simulink library "inSOMANET"  (R2016b)
settings: Solver=VariableStepAuto  StartTime=0.0  StopTime=10.0  RelTol=1e-3
undefined symbols (not defined in the file): jointPolarityLHFE, jointPolarityLKFE, jointPolarityRHFE, jointPolarityRKFE, resolutionJointEncoder, resolutionMotorEncoder, torquePolarityLHFE, torquePolarityLKFE, torquePolarityRHFE, torquePolarityRKFE, zeroOffsetLHFE, zeroOffsetLKFE, zeroOffsetRHFE, zeroOffsetRKFE
libraries: xpcethercatlib x70, ConversionsLibrary x64, simulink_extras x8
settings Model: Creator=Nathan  LastModifiedBy=march

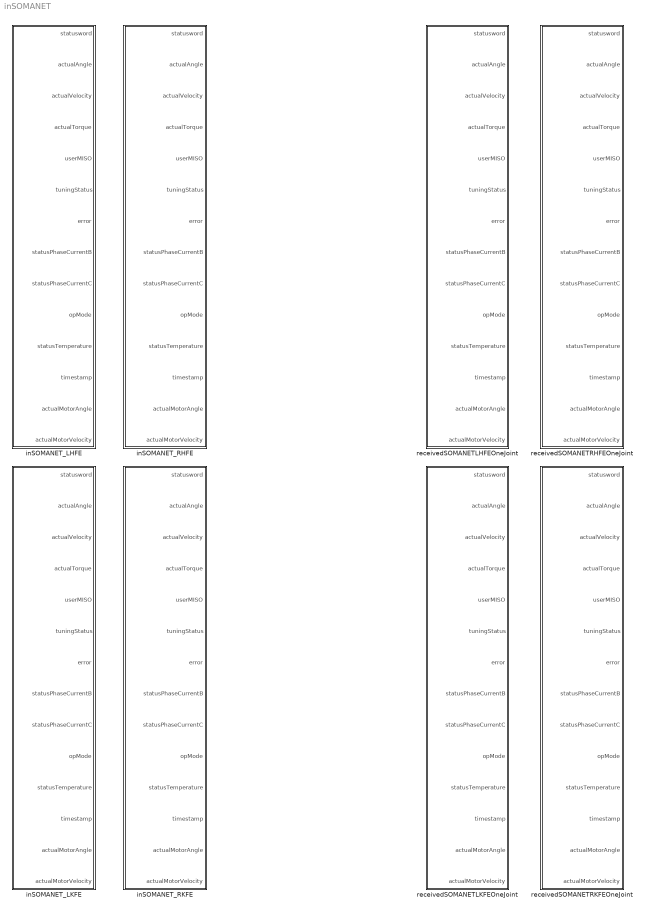
== system inSOMANET ==
  inSOMANET_LHFE : Subsystem
  inSOMANET_LKFE : Subsystem
  inSOMANET_RHFE : Subsystem
  inSOMANET_RKFE : Subsystem
  receivedSOMANETLHFEOneJoint : Subsystem
  receivedSOMANETLKFEOneJoint : Subsystem
  receivedSOMANETRHFEOneJoint : Subsystem
  receivedSOMANETRKFEOneJoint : Subsystem

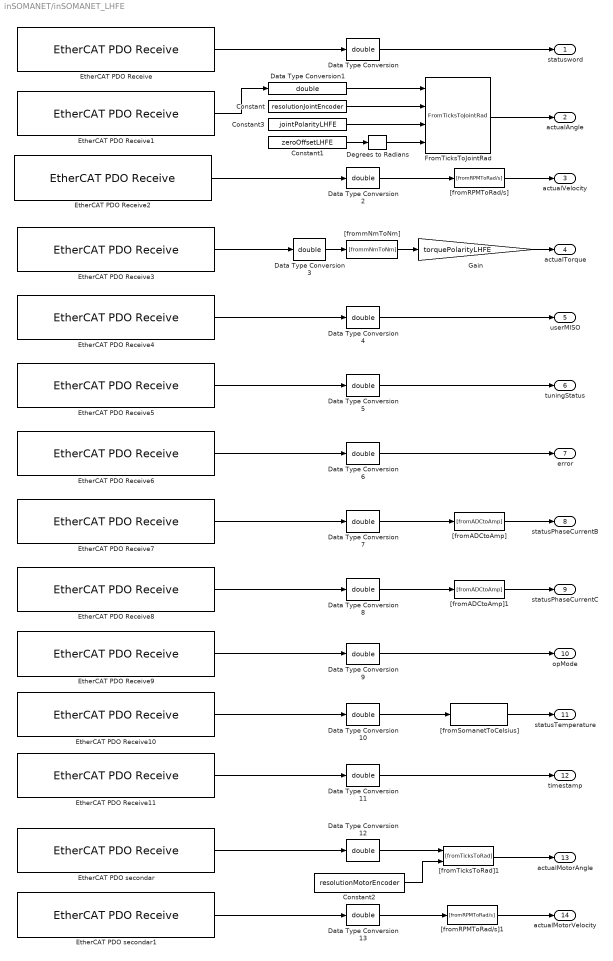
== system inSOMANET/inSOMANET_LHFE ==
  Constant : Constant  Value=resolutionJointEncoder
  Constant1 : Constant  Value=zeroOffsetLHFE  SampleTime=-1
  Constant2 : Constant  Value=resolutionMotorEncoder
  Constant3 : Constant  Value=jointPolarityLHFE
  Data Type Conversion{,1..13} (14 alike) : DataTypeConversion  OutDataTypeStr=double
  Degrees to Radians : simulink_extras/Transformations/Degrees to Radians
  EtherCAT PDO Receive : xpcethercatlib/EtherCAT PDO Receive  Priority=2  sig_name=Drive 1 LHFE.Inputs.Statusword  sig_offset=208  sig_type=uint16  type_size=16  sig_dim=1  device_id=0  sample_time=0.002000
  EtherCAT PDO Receive1 : xpcethercatlib/EtherCAT PDO Receive  Priority=2  sig_name=Drive 1 LHFE.Inputs.Position Value  sig_offset=232  sig_type=int32  type_size=32  sig_dim=1  device_id=0  sample_time=0.002000
  EtherCAT PDO Receive10 : xpcethercatlib/EtherCAT PDO Receive  Priority=2  sig_name=Drive 1 LHFE.Inputs.Core Temp  sig_offset=616  sig_type=int16  type_size=16  sig_dim=1  device_id=0  sample_time=0.002000
  EtherCAT PDO Receive11 : xpcethercatlib/EtherCAT PDO Receive  Priority=2  sig_name=Drive 1 LHFE.Inputs.timestamp  sig_offset=536  sig_type=uint32  type_size=32  sig_dim=1  device_id=0  sample_time=0.002000
  EtherCAT PDO Receive2 : xpcethercatlib/EtherCAT PDO Receive  Priority=2  sig_name=Drive 1 LHFE.Inputs.Velocity Value  sig_offset=264  sig_type=int32  type_size=32  sig_dim=1  device_id=0  sample_time=0.002000
  EtherCAT PDO Receive3 : xpcethercatlib/EtherCAT PDO Receive  Priority=2  sig_name=Drive 1 LHFE.Inputs.Torque Value  sig_offset=296  sig_type=int16  type_size=16  sig_dim=1  device_id=0  sample_time=0.002000
  EtherCAT PDO Receive4 : xpcethercatlib/EtherCAT PDO Receive  Priority=2  sig_name=Drive 1 LHFE.Inputs.User MISO  sig_offset=504  sig_type=uint32  type_size=32  sig_dim=1  device_id=0  sample_time=0.002000
  EtherCAT PDO Receive5 : xpcethercatlib/EtherCAT PDO Receive  Priority=2  sig_name=Drive 1 LHFE.Inputs.Tuning status  sig_offset=440  sig_type=uint32  type_size=32  sig_dim=1  device_id=0  sample_time=0.002000
  EtherCAT PDO Receive6 : xpcethercatlib/EtherCAT PDO Receive  Priority=2  sig_name=Drive 1 LHFE.Inputs.Error code  sig_offset=568  sig_type=uint16  type_size=16  sig_dim=1  device_id=0  sample_time=0.002000
  EtherCAT PDO Receive7 : xpcethercatlib/EtherCAT PDO Receive  Priority=2  sig_name=Drive 1 LHFE.Inputs.Phase B  sig_offset=584  sig_type=int16  type_size=16  sig_dim=1  device_id=0  sample_time=0.002000
  EtherCAT PDO Receive8 : xpcethercatlib/EtherCAT PDO Receive  Priority=2  sig_name=Drive 1 LHFE.Inputs.Phase C  sig_offset=600  sig_type=int16  type_size=16  sig_dim=1  device_id=0  sample_time=0.002000
  EtherCAT PDO Receive9 : xpcethercatlib/EtherCAT PDO Receive  Priority=2  sig_name=Drive 1 LHFE.Inputs.Op Mode Display  sig_offset=224  sig_type=int8  type_size=8  sig_dim=1  device_id=0  sample_time=0.002000
  EtherCAT PDO secondar : xpcethercatlib/EtherCAT PDO Receive  Priority=2  sig_name=Drive 1 LHFE.Inputs.Secondary position value  sig_offset=312  sig_type=int32  type_size=32  sig_dim=1  device_id=0  sample_time=0.002000
  EtherCAT PDO secondar1 : xpcethercatlib/EtherCAT PDO Receive  Priority=2  sig_name=Drive 1 LHFE.Inputs.Secondary velocity value  sig_offset=344  sig_type=int32  type_size=32  sig_dim=1  device_id=0  sample_time=0.002000
  FromTicksToJointRad : ConversionsLibrary/FromTicksToJointRad
  Gain : Gain  Gain=torquePolarityLHFE
  "[fromADCtoAmp]" : ConversionsLibrary/[fromADCtoAmp]
  "[fromADCtoAmp]1" : ConversionsLibrary/[fromADCtoAmp]
  "[fromRPMToRad/s]" : ConversionsLibrary/[fromRPMToRad//s]
  "[fromRPMToRad/s]1" : ConversionsLibrary/[fromRPMToRad//s]
  "[fromSomanetToCelsius]" : ConversionsLibrary/[fromSomanetToCelsius]
  "[fromTicksToRad]1" : ConversionsLibrary/[fromTicksToRad]
  "[frommNmToNm]" : ConversionsLibrary/[frommNmToNm]
  statusword : Outport
  actualAngle : Outport  Port=2
  actualVelocity : Outport  Port=3
  actualTorque : Outport  Port=4
  userMISO : Outport  Port=5
  tuningStatus : Outport  Port=6
  error : Outport  Port=7
  statusPhaseCurrentB : Outport  Port=8
  statusPhaseCurrentC : Outport  Port=9
  opMode : Outport  Port=10
  statusTemperature : Outport  Port=11
  timestamp : Outport  Port=12
  actualMotorAngle : Outport  Port=13
  actualMotorVelocity : Outport  Port=14
  wires:
  EtherCAT PDO secondar1/1 -> Data Type Conversion13/1
  Data Type Conversion13/1 -> "[fromRPMToRad/s]1"/1
  EtherCAT PDO secondar/1 -> Data Type Conversion12/1
  EtherCAT PDO Receive11/1 -> Data Type Conversion11/1
  EtherCAT PDO Receive10/1 -> Data Type Conversion10/1
  EtherCAT PDO Receive9/1 -> Data Type Conversion9/1
  EtherCAT PDO Receive8/1 -> Data Type Conversion8/1
  EtherCAT PDO Receive7/1 -> Data Type Conversion7/1
  EtherCAT PDO Receive6/1 -> Data Type Conversion6/1
  EtherCAT PDO Receive5/1 -> Data Type Conversion5/1
  EtherCAT PDO Receive4/1 -> Data Type Conversion4/1
  EtherCAT PDO Receive3/1 -> Data Type Conversion3/1
  EtherCAT PDO Receive2/1 -> Data Type Conversion2/1
  EtherCAT PDO Receive1/1 -> Data Type Conversion1/1
  EtherCAT PDO Receive/1 -> Data Type Conversion/1
  Data Type Conversion/1 -> statusword/1
  Data Type Conversion10/1 -> "[fromSomanetToCelsius]"/1
  Data Type Conversion9/1 -> opMode/1
  Data Type Conversion8/1 -> "[fromADCtoAmp]1"/1
  Data Type Conversion7/1 -> "[fromADCtoAmp]"/1
  Data Type Conversion6/1 -> error/1
  Data Type Conversion5/1 -> tuningStatus/1
  Data Type Conversion4/1 -> userMISO/1
  Data Type Conversion3/1 -> "[frommNmToNm]"/1
  Data Type Conversion2/1 -> "[fromRPMToRad/s]"/1
  Data Type Conversion11/1 -> timestamp/1
  "[fromSomanetToCelsius]"/1 -> statusTemperature/1
  "[fromADCtoAmp]1"/1 -> statusPhaseCurrentC/1
  "[fromADCtoAmp]"/1 -> statusPhaseCurrentB/1
  "[frommNmToNm]"/1 -> Gain/1
  "[fromRPMToRad/s]"/1 -> actualVelocity/1
  Constant1/1 -> Degrees to Radians/1
  FromTicksToJointRad/1 -> actualAngle/1
  Data Type Conversion12/1 -> "[fromTicksToRad]1"/1
  "[fromTicksToRad]1"/1 -> actualMotorAngle/1
  Constant2/1 -> "[fromTicksToRad]1"/2
  "[fromRPMToRad/s]1"/1 -> actualMotorVelocity/1
  Degrees to Radians/1 -> FromTicksToJointRad/4
  Data Type Conversion1/1 -> FromTicksToJointRad/1
  Constant/1 -> FromTicksToJointRad/2
  Constant3/1 -> FromTicksToJointRad/3
  Gain/1 -> actualTorque/1

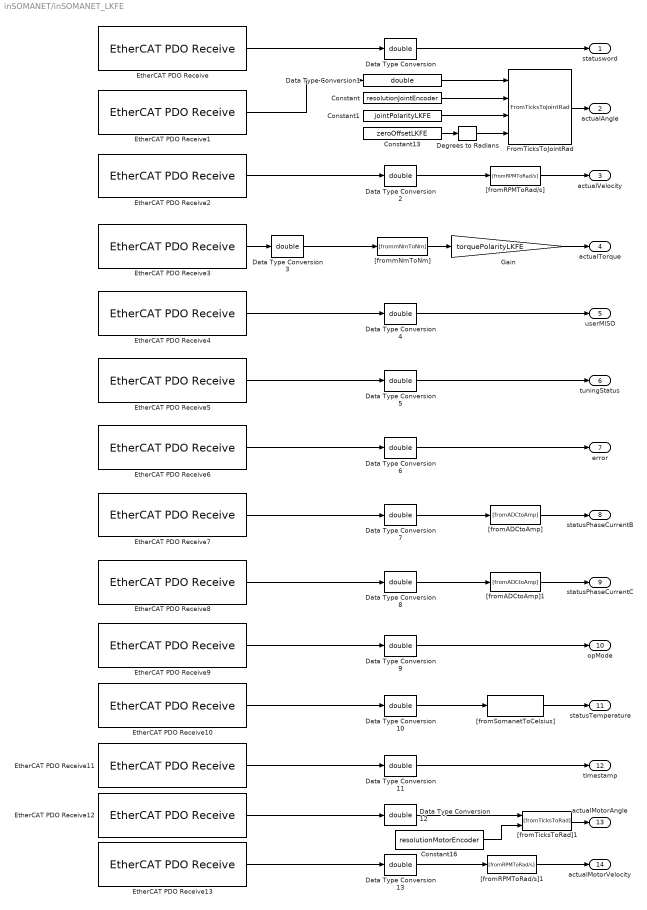
== system inSOMANET/inSOMANET_LKFE ==
  Constant : Constant  Value=resolutionJointEncoder
  Constant1 : Constant  Value=jointPolarityLKFE
  Constant13 : Constant  Value=zeroOffsetLKFE  SampleTime=-1
  Constant16 : Constant  Value=resolutionMotorEncoder
  Data Type Conversion{,1..13} (14 alike) : DataTypeConversion  OutDataTypeStr=double
  Degrees to Radians : simulink_extras/Transformations/Degrees to Radians
  EtherCAT PDO Receive : xpcethercatlib/EtherCAT PDO Receive  Priority=2  sig_name=Drive 2 LKFE.Inputs.Statusword  sig_offset=632  sig_type=uint16  type_size=16  sig_dim=1  device_id=0  sample_time=0.002000
  EtherCAT PDO Receive1 : xpcethercatlib/EtherCAT PDO Receive  Priority=2  sig_name=Drive 2 LKFE.Inputs.Position Value  sig_offset=656  sig_type=int32  type_size=32  sig_dim=1  device_id=0  sample_time=0.002000
  EtherCAT PDO Receive10 : xpcethercatlib/EtherCAT PDO Receive  Priority=2  sig_name=Drive 2 LKFE.Inputs.Core Temp  sig_offset=1040  sig_type=int16  type_size=16  sig_dim=1  device_id=0  sample_time=0.002000
  EtherCAT PDO Receive11 : xpcethercatlib/EtherCAT PDO Receive  Priority=2  sig_name=Drive 2 LKFE.Inputs.timestamp  sig_offset=960  sig_type=uint32  type_size=32  sig_dim=1  device_id=0  sample_time=0.002000
  EtherCAT PDO Receive12 : xpcethercatlib/EtherCAT PDO Receive  Priority=2  sig_name=Drive 2 LKFE.Inputs.Secondary position value  sig_offset=736  sig_type=int32  type_size=32  sig_dim=1  device_id=0  sample_time=0.002000
  EtherCAT PDO Receive13 : xpcethercatlib/EtherCAT PDO Receive  Priority=2  sig_name=Drive 2 LKFE.Inputs.Secondary velocity value  sig_offset=768  sig_type=int32  type_size=32  sig_dim=1  device_id=0  sample_time=0.002000
  EtherCAT PDO Receive2 : xpcethercatlib/EtherCAT PDO Receive  Priority=2  sig_name=Drive 2 LKFE.Inputs.Velocity Value  sig_offset=688  sig_type=int32  type_size=32  sig_dim=1  device_id=0  sample_time=0.002000
  EtherCAT PDO Receive3 : xpcethercatlib/EtherCAT PDO Receive  Priority=2  sig_name=Drive 2 LKFE.Inputs.Torque Value  sig_offset=720  sig_type=int16  type_size=16  sig_dim=1  device_id=0  sample_time=0.002000
  EtherCAT PDO Receive4 : xpcethercatlib/EtherCAT PDO Receive  Priority=2  sig_name=Drive 2 LKFE.Inputs.User MISO  sig_offset=928  sig_type=uint32  type_size=32  sig_dim=1  device_id=0  sample_time=0.002000
  EtherCAT PDO Receive5 : xpcethercatlib/EtherCAT PDO Receive  Priority=2  sig_name=Drive 2 LKFE.Inputs.Tuning status  sig_offset=864  sig_type=uint32  type_size=32  sig_dim=1  device_id=0  sample_time=0.002000
  EtherCAT PDO Receive6 : xpcethercatlib/EtherCAT PDO Receive  Priority=2  sig_name=Drive 2 LKFE.Inputs.Error code  sig_offset=992  sig_type=uint16  type_size=16  sig_dim=1  device_id=0  sample_time=0.002000
  EtherCAT PDO Receive7 : xpcethercatlib/EtherCAT PDO Receive  Priority=2  sig_name=Drive 2 LKFE.Inputs.Phase B  sig_offset=1008  sig_type=int16  type_size=16  sig_dim=1  device_id=0  sample_time=0.002000
  EtherCAT PDO Receive8 : xpcethercatlib/EtherCAT PDO Receive  Priority=2  sig_name=Drive 2 LKFE.Inputs.Phase C  sig_offset=1024  sig_type=int16  type_size=16  sig_dim=1  device_id=0  sample_time=0.002000
  EtherCAT PDO Receive9 : xpcethercatlib/EtherCAT PDO Receive  Priority=2  sig_name=Drive 2 LKFE.Inputs.Op Mode Display  sig_offset=648  sig_type=int8  type_size=8  sig_dim=1  device_id=0  sample_time=0.002000
  FromTicksToJointRad : ConversionsLibrary/FromTicksToJointRad
  Gain : Gain  Gain=torquePolarityLKFE
  "[fromADCtoAmp]" : ConversionsLibrary/[fromADCtoAmp]
  "[fromADCtoAmp]1" : ConversionsLibrary/[fromADCtoAmp]
  "[fromRPMToRad/s]" : ConversionsLibrary/[fromRPMToRad//s]
  "[fromRPMToRad/s]1" : ConversionsLibrary/[fromRPMToRad//s]
  "[fromSomanetToCelsius]" : ConversionsLibrary/[fromSomanetToCelsius]
  "[fromTicksToRad]1" : ConversionsLibrary/[fromTicksToRad]
  "[frommNmToNm]" : ConversionsLibrary/[frommNmToNm]
  statusword : Outport
  actualAngle : Outport  Port=2
  actualVelocity : Outport  Port=3
  actualTorque : Outport  Port=4
  userMISO : Outport  Port=5
  tuningStatus : Outport  Port=6
  error : Outport  Port=7
  statusPhaseCurrentB : Outport  Port=8
  statusPhaseCurrentC : Outport  Port=9
  opMode : Outport  Port=10
  statusTemperature : Outport  Port=11
  timestamp : Outport  Port=12
  actualMotorAngle : Outport  Port=13
  actualMotorVelocity : Outport  Port=14
  wires:
  EtherCAT PDO Receive13/1 -> Data Type Conversion13/1
  Data Type Conversion13/1 -> "[fromRPMToRad/s]1"/1
  EtherCAT PDO Receive12/1 -> Data Type Conversion12/1
  EtherCAT PDO Receive11/1 -> Data Type Conversion11/1
  EtherCAT PDO Receive10/1 -> Data Type Conversion10/1
  EtherCAT PDO Receive9/1 -> Data Type Conversion9/1
  EtherCAT PDO Receive8/1 -> Data Type Conversion8/1
  EtherCAT PDO Receive7/1 -> Data Type Conversion7/1
  EtherCAT PDO Receive6/1 -> Data Type Conversion6/1
  EtherCAT PDO Receive5/1 -> Data Type Conversion5/1
  EtherCAT PDO Receive4/1 -> Data Type Conversion4/1
  EtherCAT PDO Receive3/1 -> Data Type Conversion3/1
  EtherCAT PDO Receive2/1 -> Data Type Conversion2/1
  EtherCAT PDO Receive1/1 -> Data Type Conversion1/1
  EtherCAT PDO Receive/1 -> Data Type Conversion/1
  Data Type Conversion/1 -> statusword/1
  Data Type Conversion10/1 -> "[fromSomanetToCelsius]"/1
  Data Type Conversion9/1 -> opMode/1
  Data Type Conversion8/1 -> "[fromADCtoAmp]1"/1
  Data Type Conversion7/1 -> "[fromADCtoAmp]"/1
  Data Type Conversion6/1 -> error/1
  Data Type Conversion5/1 -> tuningStatus/1
  Data Type Conversion4/1 -> userMISO/1
  Data Type Conversion3/1 -> "[frommNmToNm]"/1
  Data Type Conversion2/1 -> "[fromRPMToRad/s]"/1
  Data Type Conversion11/1 -> timestamp/1
  "[fromSomanetToCelsius]"/1 -> statusTemperature/1
  "[fromADCtoAmp]1"/1 -> statusPhaseCurrentC/1
  "[fromADCtoAmp]"/1 -> statusPhaseCurrentB/1
  "[frommNmToNm]"/1 -> Gain/1
  "[fromRPMToRad/s]"/1 -> actualVelocity/1
  Constant13/1 -> Degrees to Radians/1
  Constant16/1 -> "[fromTicksToRad]1"/2
  "[fromTicksToRad]1"/1 -> actualMotorAngle/1
  Data Type Conversion12/1 -> "[fromTicksToRad]1"/1
  "[fromRPMToRad/s]1"/1 -> actualMotorVelocity/1
  Degrees to Radians/1 -> FromTicksToJointRad/4
  Constant/1 -> FromTicksToJointRad/2
  Data Type Conversion1/1 -> FromTicksToJointRad/1
  Constant1/1 -> FromTicksToJointRad/3
  FromTicksToJointRad/1 -> actualAngle/1
  Gain/1 -> actualTorque/1

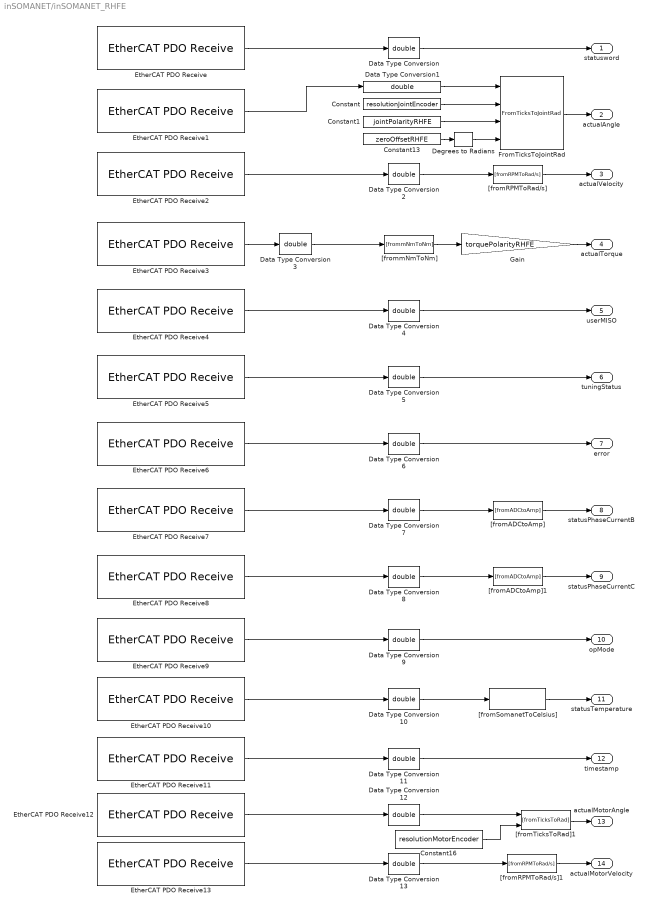
== system inSOMANET/inSOMANET_RHFE ==
  Constant : Constant  Value=resolutionJointEncoder
  Constant1 : Constant  Value=jointPolarityRHFE
  Constant13 : Constant  Value=zeroOffsetRHFE  SampleTime=-1
  Constant16 : Constant  Value=resolutionMotorEncoder
  Data Type Conversion{,1..13} (14 alike) : DataTypeConversion  OutDataTypeStr=double
  Degrees to Radians : simulink_extras/Transformations/Degrees to Radians
  EtherCAT PDO Receive : xpcethercatlib/EtherCAT PDO Receive  Priority=2  sig_name=Drive 3 RHFE.Inputs.Statusword  sig_offset=1056  sig_type=uint16  type_size=16  sig_dim=1  device_id=0  sample_time=0.002000
  EtherCAT PDO Receive1 : xpcethercatlib/EtherCAT PDO Receive  Priority=2  sig_name=Drive 3 RHFE.Inputs.Position Value  sig_offset=1080  sig_type=int32  type_size=32  sig_dim=1  device_id=0  sample_time=0.002000
  EtherCAT PDO Receive10 : xpcethercatlib/EtherCAT PDO Receive  Priority=2  sig_name=Drive 3 RHFE.Inputs.Core Temp  sig_offset=1464  sig_type=int16  type_size=16  sig_dim=1  device_id=0  sample_time=0.002000
  EtherCAT PDO Receive11 : xpcethercatlib/EtherCAT PDO Receive  Priority=2  sig_name=Drive 3 RHFE.Inputs.timestamp  sig_offset=1384  sig_type=uint32  type_size=32  sig_dim=1  device_id=0  sample_time=0.002000
  EtherCAT PDO Receive12 : xpcethercatlib/EtherCAT PDO Receive  Priority=2  sig_name=Drive 3 RHFE.Inputs.Secondary position value  sig_offset=1160  sig_type=int32  type_size=32  sig_dim=1  device_id=0  sample_time=0.002000
  EtherCAT PDO Receive13 : xpcethercatlib/EtherCAT PDO Receive  Priority=2  sig_name=Drive 3 RHFE.Inputs.Secondary velocity value  sig_offset=1192  sig_type=int32  type_size=32  sig_dim=1  device_id=0  sample_time=0.002000
  EtherCAT PDO Receive2 : xpcethercatlib/EtherCAT PDO Receive  Priority=2  sig_name=Drive 3 RHFE.Inputs.Velocity Value  sig_offset=1112  sig_type=int32  type_size=32  sig_dim=1  device_id=0  sample_time=0.002000
  EtherCAT PDO Receive3 : xpcethercatlib/EtherCAT PDO Receive  Priority=2  sig_name=Drive 3 RHFE.Inputs.Torque Value  sig_offset=1144  sig_type=int16  type_size=16  sig_dim=1  device_id=0  sample_time=0.002000
  EtherCAT PDO Receive4 : xpcethercatlib/EtherCAT PDO Receive  Priority=2  sig_name=Drive 3 RHFE.Inputs.User MISO  sig_offset=1352  sig_type=uint32  type_size=32  sig_dim=1  device_id=0  sample_time=0.002000
  EtherCAT PDO Receive5 : xpcethercatlib/EtherCAT PDO Receive  Priority=2  sig_name=Drive 3 RHFE.Inputs.Tuning status  sig_offset=1288  sig_type=uint32  type_size=32  sig_dim=1  device_id=0  sample_time=0.002000
  EtherCAT PDO Receive6 : xpcethercatlib/EtherCAT PDO Receive  Priority=2  sig_name=Drive 3 RHFE.Inputs.Error code  sig_offset=1416  sig_type=uint16  type_size=16  sig_dim=1  device_id=0  sample_time=0.002000
  EtherCAT PDO Receive7 : xpcethercatlib/EtherCAT PDO Receive  Priority=2  sig_name=Drive 3 RHFE.Inputs.Phase B  sig_offset=1432  sig_type=int16  type_size=16  sig_dim=1  device_id=0  sample_time=0.002000
  EtherCAT PDO Receive8 : xpcethercatlib/EtherCAT PDO Receive  Priority=2  sig_name=Drive 3 RHFE.Inputs.Phase C  sig_offset=1448  sig_type=int16  type_size=16  sig_dim=1  device_id=0  sample_time=0.002000
  EtherCAT PDO Receive9 : xpcethercatlib/EtherCAT PDO Receive  Priority=2  sig_name=Drive 3 RHFE.Inputs.Op Mode Display  sig_offset=1072  sig_type=int8  type_size=8  sig_dim=1  device_id=0  sample_time=0.002000
  FromTicksToJointRad : ConversionsLibrary/FromTicksToJointRad
  Gain : Gain  Gain=torquePolarityRHFE
  "[fromADCtoAmp]" : ConversionsLibrary/[fromADCtoAmp]
  "[fromADCtoAmp]1" : ConversionsLibrary/[fromADCtoAmp]
  "[fromRPMToRad/s]" : ConversionsLibrary/[fromRPMToRad//s]
  "[fromRPMToRad/s]1" : ConversionsLibrary/[fromRPMToRad//s]
  "[fromSomanetToCelsius]" : ConversionsLibrary/[fromSomanetToCelsius]
  "[fromTicksToRad]1" : ConversionsLibrary/[fromTicksToRad]
  "[frommNmToNm]" : ConversionsLibrary/[frommNmToNm]
  statusword : Outport
  actualAngle : Outport  Port=2
  actualVelocity : Outport  Port=3
  actualTorque : Outport  Port=4
  userMISO : Outport  Port=5
  tuningStatus : Outport  Port=6
  error : Outport  Port=7
  statusPhaseCurrentB : Outport  Port=8
  statusPhaseCurrentC : Outport  Port=9
  opMode : Outport  Port=10
  statusTemperature : Outport  Port=11
  timestamp : Outport  Port=12
  actualMotorAngle : Outport  Port=13
  actualMotorVelocity : Outport  Port=14
  wires:
  EtherCAT PDO Receive13/1 -> Data Type Conversion13/1
  Data Type Conversion13/1 -> "[fromRPMToRad/s]1"/1
  EtherCAT PDO Receive12/1 -> Data Type Conversion12/1
  EtherCAT PDO Receive11/1 -> Data Type Conversion11/1
  EtherCAT PDO Receive10/1 -> Data Type Conversion10/1
  EtherCAT PDO Receive9/1 -> Data Type Conversion9/1
  EtherCAT PDO Receive8/1 -> Data Type Conversion8/1
  EtherCAT PDO Receive7/1 -> Data Type Conversion7/1
  EtherCAT PDO Receive6/1 -> Data Type Conversion6/1
  EtherCAT PDO Receive5/1 -> Data Type Conversion5/1
  EtherCAT PDO Receive4/1 -> Data Type Conversion4/1
  EtherCAT PDO Receive3/1 -> Data Type Conversion3/1
  EtherCAT PDO Receive2/1 -> Data Type Conversion2/1
  EtherCAT PDO Receive1/1 -> Data Type Conversion1/1
  EtherCAT PDO Receive/1 -> Data Type Conversion/1
  Data Type Conversion/1 -> statusword/1
  Data Type Conversion10/1 -> "[fromSomanetToCelsius]"/1
  Data Type Conversion9/1 -> opMode/1
  Data Type Conversion8/1 -> "[fromADCtoAmp]1"/1
  Data Type Conversion7/1 -> "[fromADCtoAmp]"/1
  Data Type Conversion6/1 -> error/1
  Data Type Conversion5/1 -> tuningStatus/1
  Data Type Conversion4/1 -> userMISO/1
  Data Type Conversion3/1 -> "[frommNmToNm]"/1
  Data Type Conversion2/1 -> "[fromRPMToRad/s]"/1
  Data Type Conversion11/1 -> timestamp/1
  "[fromSomanetToCelsius]"/1 -> statusTemperature/1
  "[fromADCtoAmp]1"/1 -> statusPhaseCurrentC/1
  "[fromADCtoAmp]"/1 -> statusPhaseCurrentB/1
  "[frommNmToNm]"/1 -> Gain/1
  "[fromRPMToRad/s]"/1 -> actualVelocity/1
  Constant13/1 -> Degrees to Radians/1
  FromTicksToJointRad/1 -> actualAngle/1
  Constant16/1 -> "[fromTicksToRad]1"/2
  "[fromTicksToRad]1"/1 -> actualMotorAngle/1
  Data Type Conversion12/1 -> "[fromTicksToRad]1"/1
  "[fromRPMToRad/s]1"/1 -> actualMotorVelocity/1
  Data Type Conversion1/1 -> FromTicksToJointRad/1
  Constant/1 -> FromTicksToJointRad/2
  Constant1/1 -> FromTicksToJointRad/3
  Degrees to Radians/1 -> FromTicksToJointRad/4
  Gain/1 -> actualTorque/1

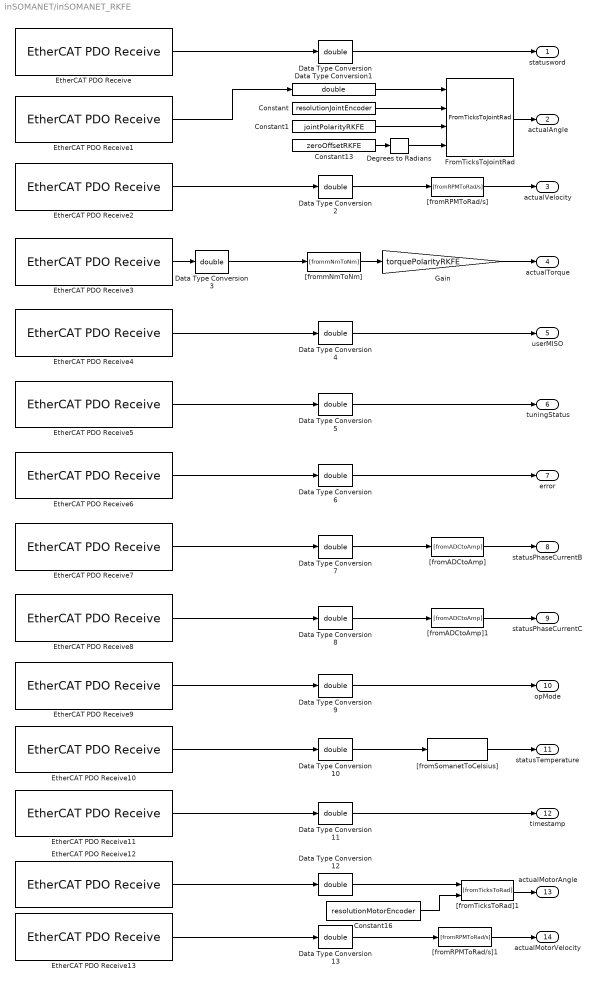
== system inSOMANET/inSOMANET_RKFE ==
  Constant : Constant  Value=resolutionJointEncoder
  Constant1 : Constant  Value=jointPolarityRKFE
  Constant13 : Constant  Value=zeroOffsetRKFE  SampleTime=-1
  Constant16 : Constant  Value=resolutionMotorEncoder
  Data Type Conversion{,1..13} (14 alike) : DataTypeConversion  OutDataTypeStr=double
  Degrees to Radians : simulink_extras/Transformations/Degrees to Radians
  EtherCAT PDO Receive : xpcethercatlib/EtherCAT PDO Receive  Priority=2  sig_name=Drive 4 RKFE.Inputs.Statusword  sig_offset=1480  sig_type=uint16  type_size=16  sig_dim=1  device_id=0  sample_time=0.002000
  EtherCAT PDO Receive1 : xpcethercatlib/EtherCAT PDO Receive  Priority=2  sig_name=Drive 4 RKFE.Inputs.Position Value  sig_offset=1504  sig_type=int32  type_size=32  sig_dim=1  device_id=0  sample_time=0.002000
  EtherCAT PDO Receive10 : xpcethercatlib/EtherCAT PDO Receive  Priority=2  sig_name=Drive 4 RKFE.Inputs.Core Temp  sig_offset=1888  sig_type=int16  type_size=16  sig_dim=1  device_id=0  sample_time=0.002000
  EtherCAT PDO Receive11 : xpcethercatlib/EtherCAT PDO Receive  Priority=2  sig_name=Drive 4 RKFE.Inputs.timestamp  sig_offset=1808  sig_type=uint32  type_size=32  sig_dim=1  device_id=0  sample_time=0.002000
  EtherCAT PDO Receive12 : xpcethercatlib/EtherCAT PDO Receive  Priority=2  sig_name=Drive 4 RKFE.Inputs.Secondary position value  sig_offset=1584  sig_type=int32  type_size=32  sig_dim=1  device_id=0  sample_time=0.002000
  EtherCAT PDO Receive13 : xpcethercatlib/EtherCAT PDO Receive  Priority=2  sig_name=Drive 4 RKFE.Inputs.Secondary velocity value  sig_offset=1616  sig_type=int32  type_size=32  sig_dim=1  device_id=0  sample_time=0.002000
  EtherCAT PDO Receive2 : xpcethercatlib/EtherCAT PDO Receive  Priority=2  sig_name=Drive 4 RKFE.Inputs.Velocity Value  sig_offset=1536  sig_type=int32  type_size=32  sig_dim=1  device_id=0  sample_time=0.002000
  EtherCAT PDO Receive3 : xpcethercatlib/EtherCAT PDO Receive  Priority=2  sig_name=Drive 4 RKFE.Inputs.Torque Value  sig_offset=1568  sig_type=int16  type_size=16  sig_dim=1  device_id=0  sample_time=0.002000
  EtherCAT PDO Receive4 : xpcethercatlib/EtherCAT PDO Receive  Priority=2  sig_name=Drive 4 RKFE.Inputs.User MISO  sig_offset=1776  sig_type=uint32  type_size=32  sig_dim=1  device_id=0  sample_time=0.002000
  EtherCAT PDO Receive5 : xpcethercatlib/EtherCAT PDO Receive  Priority=2  sig_name=Drive 4 RKFE.Inputs.Tuning status  sig_offset=1712  sig_type=uint32  type_size=32  sig_dim=1  device_id=0  sample_time=0.002000
  EtherCAT PDO Receive6 : xpcethercatlib/EtherCAT PDO Receive  Priority=2  sig_name=Drive 4 RKFE.Inputs.Error code  sig_offset=1840  sig_type=uint16  type_size=16  sig_dim=1  device_id=0  sample_time=0.002000
  EtherCAT PDO Receive7 : xpcethercatlib/EtherCAT PDO Receive  Priority=2  sig_name=Drive 4 RKFE.Inputs.Phase B  sig_offset=1856  sig_type=int16  type_size=16  sig_dim=1  device_id=0  sample_time=0.002000
  EtherCAT PDO Receive8 : xpcethercatlib/EtherCAT PDO Receive  Priority=2  sig_name=Drive 4 RKFE.Inputs.Phase C  sig_offset=1872  sig_type=int16  type_size=16  sig_dim=1  device_id=0  sample_time=0.002000
  EtherCAT PDO Receive9 : xpcethercatlib/EtherCAT PDO Receive  Priority=2  sig_name=Drive 4 RKFE.Inputs.Op Mode Display  sig_offset=1496  sig_type=int8  type_size=8  sig_dim=1  device_id=0  sample_time=0.002000
  FromTicksToJointRad : ConversionsLibrary/FromTicksToJointRad
  Gain : Gain  Gain=torquePolarityRKFE
  "[fromADCtoAmp]" : ConversionsLibrary/[fromADCtoAmp]
  "[fromADCtoAmp]1" : ConversionsLibrary/[fromADCtoAmp]
  "[fromRPMToRad/s]" : ConversionsLibrary/[fromRPMToRad//s]
  "[fromRPMToRad/s]1" : ConversionsLibrary/[fromRPMToRad//s]
  "[fromSomanetToCelsius]" : ConversionsLibrary/[fromSomanetToCelsius]
  "[fromTicksToRad]1" : ConversionsLibrary/[fromTicksToRad]
  "[frommNmToNm]" : ConversionsLibrary/[frommNmToNm]
  statusword : Outport
  actualAngle : Outport  Port=2
  actualVelocity : Outport  Port=3
  actualTorque : Outport  Port=4
  userMISO : Outport  Port=5
  tuningStatus : Outport  Port=6
  error : Outport  Port=7
  statusPhaseCurrentB : Outport  Port=8
  statusPhaseCurrentC : Outport  Port=9
  opMode : Outport  Port=10
  statusTemperature : Outport  Port=11
  timestamp : Outport  Port=12
  actualMotorAngle : Outport  Port=13
  actualMotorVelocity : Outport  Port=14
  wires:
  EtherCAT PDO Receive13/1 -> Data Type Conversion13/1
  Data Type Conversion13/1 -> "[fromRPMToRad/s]1"/1
  EtherCAT PDO Receive12/1 -> Data Type Conversion12/1
  EtherCAT PDO Receive11/1 -> Data Type Conversion11/1
  EtherCAT PDO Receive10/1 -> Data Type Conversion10/1
  EtherCAT PDO Receive9/1 -> Data Type Conversion9/1
  EtherCAT PDO Receive8/1 -> Data Type Conversion8/1
  EtherCAT PDO Receive7/1 -> Data Type Conversion7/1
  EtherCAT PDO Receive6/1 -> Data Type Conversion6/1
  EtherCAT PDO Receive5/1 -> Data Type Conversion5/1
  EtherCAT PDO Receive4/1 -> Data Type Conversion4/1
  EtherCAT PDO Receive3/1 -> Data Type Conversion3/1
  EtherCAT PDO Receive2/1 -> Data Type Conversion2/1
  EtherCAT PDO Receive1/1 -> Data Type Conversion1/1
  EtherCAT PDO Receive/1 -> Data Type Conversion/1
  Data Type Conversion/1 -> statusword/1
  Data Type Conversion10/1 -> "[fromSomanetToCelsius]"/1
  Data Type Conversion9/1 -> opMode/1
  Data Type Conversion8/1 -> "[fromADCtoAmp]1"/1
  Data Type Conversion7/1 -> "[fromADCtoAmp]"/1
  Data Type Conversion6/1 -> error/1
  Data Type Conversion5/1 -> tuningStatus/1
  Data Type Conversion4/1 -> userMISO/1
  Data Type Conversion3/1 -> "[frommNmToNm]"/1
  Data Type Conversion2/1 -> "[fromRPMToRad/s]"/1
  Data Type Conversion11/1 -> timestamp/1
  "[fromSomanetToCelsius]"/1 -> statusTemperature/1
  "[fromADCtoAmp]1"/1 -> statusPhaseCurrentC/1
  "[fromADCtoAmp]"/1 -> statusPhaseCurrentB/1
  "[frommNmToNm]"/1 -> Gain/1
  "[fromRPMToRad/s]"/1 -> actualVelocity/1
  Constant13/1 -> Degrees to Radians/1
  Constant16/1 -> "[fromTicksToRad]1"/2
  "[fromTicksToRad]1"/1 -> actualMotorAngle/1
  Data Type Conversion12/1 -> "[fromTicksToRad]1"/1
  "[fromRPMToRad/s]1"/1 -> actualMotorVelocity/1
  Degrees to Radians/1 -> FromTicksToJointRad/4
  Data Type Conversion1/1 -> FromTicksToJointRad/1
  Constant/1 -> FromTicksToJointRad/2
  Constant1/1 -> FromTicksToJointRad/3
  FromTicksToJointRad/1 -> actualAngle/1
  Gain/1 -> actualTorque/1

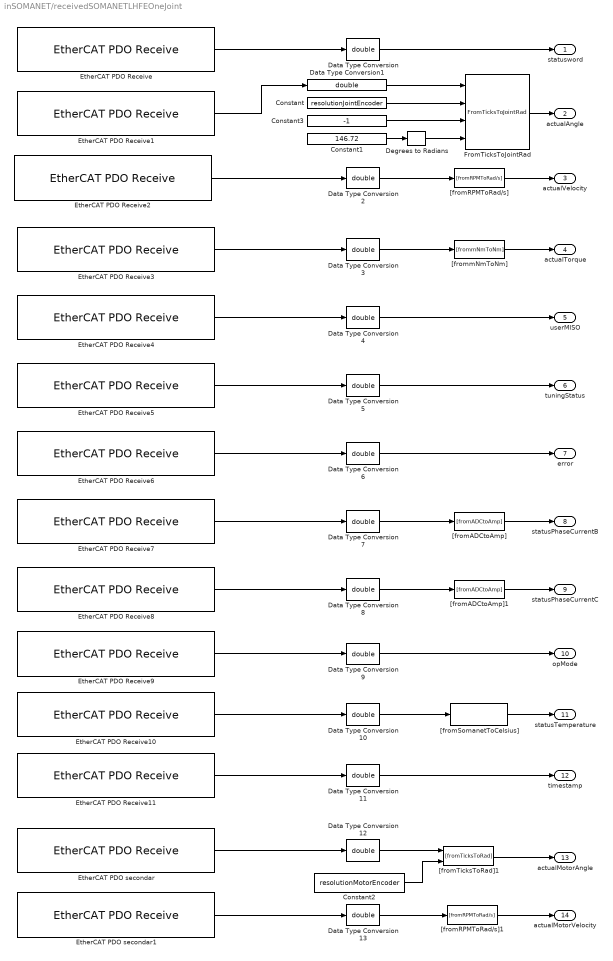
== system inSOMANET/receivedSOMANETLHFEOneJoint ==
  Constant : Constant  Value=resolutionJointEncoder
  Constant1 : Constant  Value=146.72  SampleTime=-1
  Constant2 : Constant  Value=resolutionMotorEncoder
  Constant3 : Constant  Value=-1
  Data Type Conversion{,1..13} (14 alike) : DataTypeConversion  OutDataTypeStr=double
  Degrees to Radians : simulink_extras/Transformations/Degrees to Radians
  EtherCAT PDO Receive : xpcethercatlib/EtherCAT PDO Receive  Priority=2  sig_name=Drive 1 LHFE.Inputs.Statusword  sig_offset=208  sig_type=uint16  type_size=16  sig_dim=1  device_id=0  sample_time=0.002000
  EtherCAT PDO Receive1 : xpcethercatlib/EtherCAT PDO Receive  Priority=2  sig_name=Drive 1 LHFE.Inputs.Position Value  sig_offset=232  sig_type=int32  type_size=32  sig_dim=1  device_id=0  sample_time=0.002000
  EtherCAT PDO Receive10 : xpcethercatlib/EtherCAT PDO Receive  Priority=2  sig_name=Drive 1 LHFE.Inputs.Core Temp  sig_offset=616  sig_type=int16  type_size=16  sig_dim=1  device_id=0  sample_time=0.002000
  EtherCAT PDO Receive11 : xpcethercatlib/EtherCAT PDO Receive  Priority=2  sig_name=Drive 1 LHFE.Inputs.timestamp  sig_offset=536  sig_type=uint32  type_size=32  sig_dim=1  device_id=0  sample_time=0.002000
  EtherCAT PDO Receive2 : xpcethercatlib/EtherCAT PDO Receive  Priority=2  sig_name=Drive 1 LHFE.Inputs.Velocity Value  sig_offset=264  sig_type=int32  type_size=32  sig_dim=1  device_id=0  sample_time=0.002000
  EtherCAT PDO Receive3 : xpcethercatlib/EtherCAT PDO Receive  Priority=2  sig_name=Drive 1 LHFE.Inputs.Torque Value  sig_offset=296  sig_type=int16  type_size=16  sig_dim=1  device_id=0  sample_time=0.002000
  EtherCAT PDO Receive4 : xpcethercatlib/EtherCAT PDO Receive  Priority=2  sig_name=Drive 1 LHFE.Inputs.User MISO  sig_offset=504  sig_type=uint32  type_size=32  sig_dim=1  device_id=0  sample_time=0.002000
  EtherCAT PDO Receive5 : xpcethercatlib/EtherCAT PDO Receive  Priority=2  sig_name=Drive 1 LHFE.Inputs.Tuning status  sig_offset=440  sig_type=uint32  type_size=32  sig_dim=1  device_id=0  sample_time=0.002000
  EtherCAT PDO Receive6 : xpcethercatlib/EtherCAT PDO Receive  Priority=2  sig_name=Drive 1 LHFE.Inputs.Error code  sig_offset=568  sig_type=uint16  type_size=16  sig_dim=1  device_id=0  sample_time=0.002000
  EtherCAT PDO Receive7 : xpcethercatlib/EtherCAT PDO Receive  Priority=2  sig_name=Drive 1 LHFE.Inputs.Phase B  sig_offset=584  sig_type=int16  type_size=16  sig_dim=1  device_id=0  sample_time=0.002000
  EtherCAT PDO Receive8 : xpcethercatlib/EtherCAT PDO Receive  Priority=2  sig_name=Drive 1 LHFE.Inputs.Phase C  sig_offset=600  sig_type=int16  type_size=16  sig_dim=1  device_id=0  sample_time=0.002000
  EtherCAT PDO Receive9 : xpcethercatlib/EtherCAT PDO Receive  Priority=2  sig_name=Drive 1 LHFE.Inputs.Op Mode Display  sig_offset=224  sig_type=int8  type_size=8  sig_dim=1  device_id=0  sample_time=0.002000
  EtherCAT PDO secondar : xpcethercatlib/EtherCAT PDO Receive  Priority=2  sig_name=Drive 1 LHFE.Inputs.Secondary position value  sig_offset=312  sig_type=int32  type_size=32  sig_dim=1  device_id=0  sample_time=0.002000
  EtherCAT PDO secondar1 : xpcethercatlib/EtherCAT PDO Receive  Priority=2  sig_name=Drive 1 LHFE.Inputs.Secondary velocity value  sig_offset=344  sig_type=int32  type_size=32  sig_dim=1  device_id=0  sample_time=0.002000
  FromTicksToJointRad : ConversionsLibrary/FromTicksToJointRad
  "[fromADCtoAmp]" : ConversionsLibrary/[fromADCtoAmp]
  "[fromADCtoAmp]1" : ConversionsLibrary/[fromADCtoAmp]
  "[fromRPMToRad/s]" : ConversionsLibrary/[fromRPMToRad//s]
  "[fromRPMToRad/s]1" : ConversionsLibrary/[fromRPMToRad//s]
  "[fromSomanetToCelsius]" : ConversionsLibrary/[fromSomanetToCelsius]
  "[fromTicksToRad]1" : ConversionsLibrary/[fromTicksToRad]
  "[frommNmToNm]" : ConversionsLibrary/[frommNmToNm]
  statusword : Outport
  actualAngle : Outport  Port=2
  actualVelocity : Outport  Port=3
  actualTorque : Outport  Port=4
  userMISO : Outport  Port=5
  tuningStatus : Outport  Port=6
  error : Outport  Port=7
  statusPhaseCurrentB : Outport  Port=8
  statusPhaseCurrentC : Outport  Port=9
  opMode : Outport  Port=10
  statusTemperature : Outport  Port=11
  timestamp : Outport  Port=12
  actualMotorAngle : Outport  Port=13
  actualMotorVelocity : Outport  Port=14
  wires:
  EtherCAT PDO secondar1/1 -> Data Type Conversion13/1
  Data Type Conversion13/1 -> "[fromRPMToRad/s]1"/1
  EtherCAT PDO secondar/1 -> Data Type Conversion12/1
  EtherCAT PDO Receive11/1 -> Data Type Conversion11/1
  EtherCAT PDO Receive10/1 -> Data Type Conversion10/1
  EtherCAT PDO Receive9/1 -> Data Type Conversion9/1
  EtherCAT PDO Receive8/1 -> Data Type Conversion8/1
  EtherCAT PDO Receive7/1 -> Data Type Conversion7/1
  EtherCAT PDO Receive6/1 -> Data Type Conversion6/1
  EtherCAT PDO Receive5/1 -> Data Type Conversion5/1
  EtherCAT PDO Receive4/1 -> Data Type Conversion4/1
  EtherCAT PDO Receive3/1 -> Data Type Conversion3/1
  EtherCAT PDO Receive2/1 -> Data Type Conversion2/1
  EtherCAT PDO Receive1/1 -> Data Type Conversion1/1
  EtherCAT PDO Receive/1 -> Data Type Conversion/1
  Data Type Conversion/1 -> statusword/1
  Data Type Conversion10/1 -> "[fromSomanetToCelsius]"/1
  Data Type Conversion9/1 -> opMode/1
  Data Type Conversion8/1 -> "[fromADCtoAmp]1"/1
  Data Type Conversion7/1 -> "[fromADCtoAmp]"/1
  Data Type Conversion6/1 -> error/1
  Data Type Conversion5/1 -> tuningStatus/1
  Data Type Conversion4/1 -> userMISO/1
  Data Type Conversion3/1 -> "[frommNmToNm]"/1
  Data Type Conversion2/1 -> "[fromRPMToRad/s]"/1
  Data Type Conversion11/1 -> timestamp/1
  "[fromSomanetToCelsius]"/1 -> statusTemperature/1
  "[fromADCtoAmp]1"/1 -> statusPhaseCurrentC/1
  "[fromADCtoAmp]"/1 -> statusPhaseCurrentB/1
  "[frommNmToNm]"/1 -> actualTorque/1
  "[fromRPMToRad/s]"/1 -> actualVelocity/1
  Data Type Conversion12/1 -> "[fromTicksToRad]1"/1
  "[fromTicksToRad]1"/1 -> actualMotorAngle/1
  Constant2/1 -> "[fromTicksToRad]1"/2
  "[fromRPMToRad/s]1"/1 -> actualMotorVelocity/1
  Constant1/1 -> Degrees to Radians/1
  FromTicksToJointRad/1 -> actualAngle/1
  Degrees to Radians/1 -> FromTicksToJointRad/4
  Data Type Conversion1/1 -> FromTicksToJointRad/1
  Constant/1 -> FromTicksToJointRad/2
  Constant3/1 -> FromTicksToJointRad/3

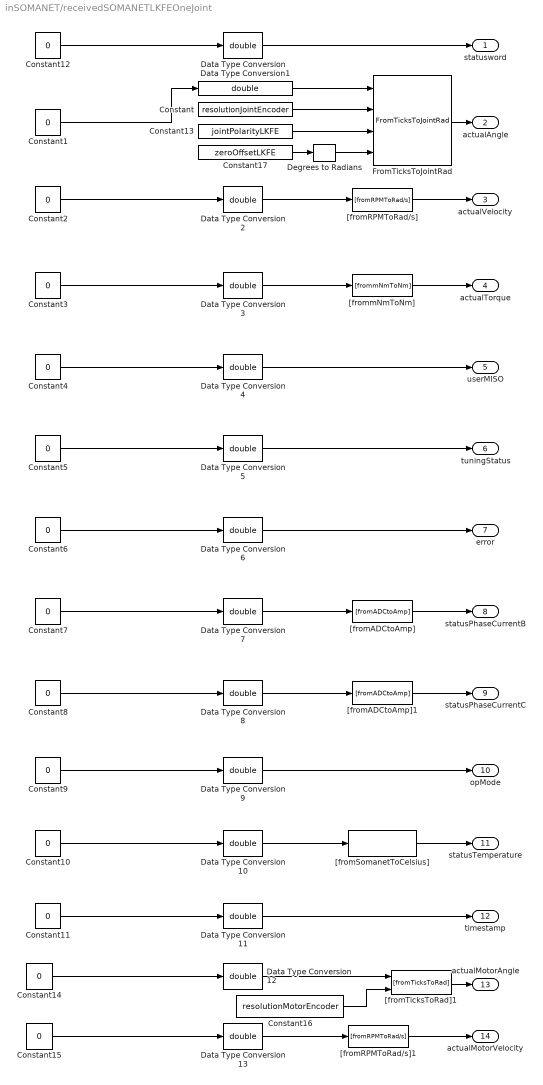
== system inSOMANET/receivedSOMANETLKFEOneJoint ==
  Constant : Constant  Value=resolutionJointEncoder
  Constant{1..12,14..15} (14 alike) : Constant  Value=0
  Constant13 : Constant  Value=jointPolarityLKFE
  Constant16 : Constant  Value=resolutionMotorEncoder
  Constant17 : Constant  Value=zeroOffsetLKFE  SampleTime=-1
  Data Type Conversion{,1..13} (14 alike) : DataTypeConversion  OutDataTypeStr=double
  Degrees to Radians : simulink_extras/Transformations/Degrees to Radians
  FromTicksToJointRad : ConversionsLibrary/FromTicksToJointRad
  "[fromADCtoAmp]" : ConversionsLibrary/[fromADCtoAmp]
  "[fromADCtoAmp]1" : ConversionsLibrary/[fromADCtoAmp]
  "[fromRPMToRad/s]" : ConversionsLibrary/[fromRPMToRad//s]
  "[fromRPMToRad/s]1" : ConversionsLibrary/[fromRPMToRad//s]
  "[fromSomanetToCelsius]" : ConversionsLibrary/[fromSomanetToCelsius]
  "[fromTicksToRad]1" : ConversionsLibrary/[fromTicksToRad]
  "[frommNmToNm]" : ConversionsLibrary/[frommNmToNm]
  statusword : Outport
  actualAngle : Outport  Port=2
  actualVelocity : Outport  Port=3
  actualTorque : Outport  Port=4
  userMISO : Outport  Port=5
  tuningStatus : Outport  Port=6
  error : Outport  Port=7
  statusPhaseCurrentB : Outport  Port=8
  statusPhaseCurrentC : Outport  Port=9
  opMode : Outport  Port=10
  statusTemperature : Outport  Port=11
  timestamp : Outport  Port=12
  actualMotorAngle : Outport  Port=13
  actualMotorVelocity : Outport  Port=14
  wires:
  Constant15/1 -> Data Type Conversion13/1
  Data Type Conversion13/1 -> "[fromRPMToRad/s]1"/1
  Constant14/1 -> Data Type Conversion12/1
  Constant11/1 -> Data Type Conversion11/1
  Constant10/1 -> Data Type Conversion10/1
  Constant9/1 -> Data Type Conversion9/1
  Constant8/1 -> Data Type Conversion8/1
  Constant7/1 -> Data Type Conversion7/1
  Constant6/1 -> Data Type Conversion6/1
  Constant5/1 -> Data Type Conversion5/1
  Constant4/1 -> Data Type Conversion4/1
  Constant3/1 -> Data Type Conversion3/1
  Constant2/1 -> Data Type Conversion2/1
  Constant1/1 -> Data Type Conversion1/1
  Constant12/1 -> Data Type Conversion/1
  Data Type Conversion/1 -> statusword/1
  Data Type Conversion10/1 -> "[fromSomanetToCelsius]"/1
  Data Type Conversion9/1 -> opMode/1
  Data Type Conversion8/1 -> "[fromADCtoAmp]1"/1
  Data Type Conversion7/1 -> "[fromADCtoAmp]"/1
  Data Type Conversion6/1 -> error/1
  Data Type Conversion5/1 -> tuningStatus/1
  Data Type Conversion4/1 -> userMISO/1
  Data Type Conversion3/1 -> "[frommNmToNm]"/1
  Data Type Conversion2/1 -> "[fromRPMToRad/s]"/1
  Data Type Conversion11/1 -> timestamp/1
  "[fromSomanetToCelsius]"/1 -> statusTemperature/1
  "[fromADCtoAmp]1"/1 -> statusPhaseCurrentC/1
  "[fromADCtoAmp]"/1 -> statusPhaseCurrentB/1
  "[frommNmToNm]"/1 -> actualTorque/1
  "[fromRPMToRad/s]"/1 -> actualVelocity/1
  Constant16/1 -> "[fromTicksToRad]1"/2
  "[fromTicksToRad]1"/1 -> actualMotorAngle/1
  Data Type Conversion12/1 -> "[fromTicksToRad]1"/1
  "[fromRPMToRad/s]1"/1 -> actualMotorVelocity/1
  Constant17/1 -> Degrees to Radians/1
  Degrees to Radians/1 -> FromTicksToJointRad/4
  Constant/1 -> FromTicksToJointRad/2
  Data Type Conversion1/1 -> FromTicksToJointRad/1
  Constant13/1 -> FromTicksToJointRad/3
  FromTicksToJointRad/1 -> actualAngle/1

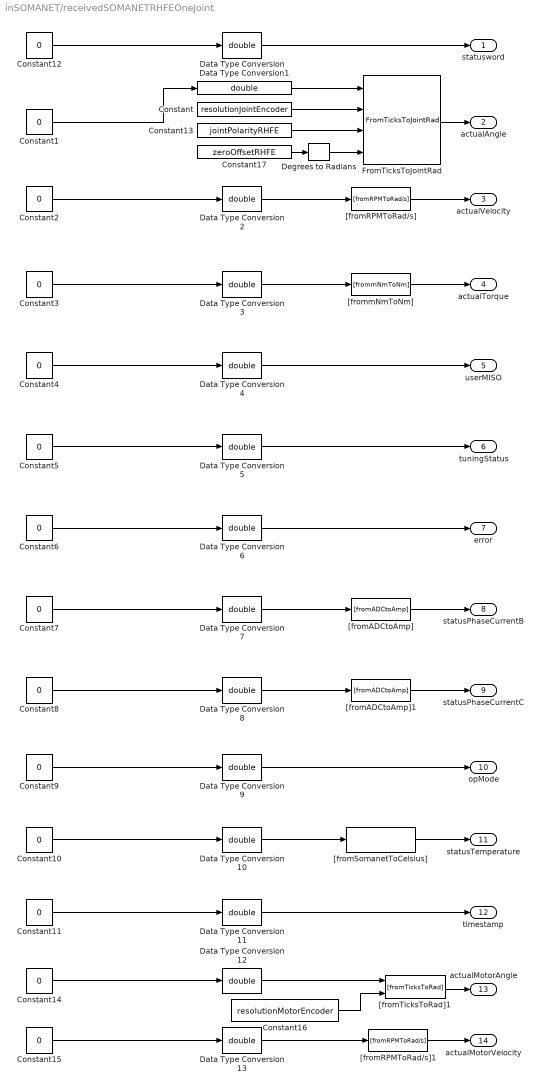
== system inSOMANET/receivedSOMANETRHFEOneJoint ==
  Constant : Constant  Value=resolutionJointEncoder
  Constant{1..12,14..15} (14 alike) : Constant  Value=0
  Constant13 : Constant  Value=jointPolarityRHFE
  Constant16 : Constant  Value=resolutionMotorEncoder
  Constant17 : Constant  Value=zeroOffsetRHFE  SampleTime=-1
  Data Type Conversion{,1..13} (14 alike) : DataTypeConversion  OutDataTypeStr=double
  Degrees to Radians : simulink_extras/Transformations/Degrees to Radians
  FromTicksToJointRad : ConversionsLibrary/FromTicksToJointRad
  "[fromADCtoAmp]" : ConversionsLibrary/[fromADCtoAmp]
  "[fromADCtoAmp]1" : ConversionsLibrary/[fromADCtoAmp]
  "[fromRPMToRad/s]" : ConversionsLibrary/[fromRPMToRad//s]
  "[fromRPMToRad/s]1" : ConversionsLibrary/[fromRPMToRad//s]
  "[fromSomanetToCelsius]" : ConversionsLibrary/[fromSomanetToCelsius]
  "[fromTicksToRad]1" : ConversionsLibrary/[fromTicksToRad]
  "[frommNmToNm]" : ConversionsLibrary/[frommNmToNm]
  statusword : Outport
  actualAngle : Outport  Port=2
  actualVelocity : Outport  Port=3
  actualTorque : Outport  Port=4
  userMISO : Outport  Port=5
  tuningStatus : Outport  Port=6
  error : Outport  Port=7
  statusPhaseCurrentB : Outport  Port=8
  statusPhaseCurrentC : Outport  Port=9
  opMode : Outport  Port=10
  statusTemperature : Outport  Port=11
  timestamp : Outport  Port=12
  actualMotorAngle : Outport  Port=13
  actualMotorVelocity : Outport  Port=14
  wires:
  Degrees to Radians/1 -> FromTicksToJointRad/4
  Constant13/1 -> FromTicksToJointRad/3
  Constant15/1 -> Data Type Conversion13/1
  Data Type Conversion13/1 -> "[fromRPMToRad/s]1"/1
  Constant14/1 -> Data Type Conversion12/1
  Constant11/1 -> Data Type Conversion11/1
  Constant10/1 -> Data Type Conversion10/1
  Constant9/1 -> Data Type Conversion9/1
  Constant8/1 -> Data Type Conversion8/1
  Constant7/1 -> Data Type Conversion7/1
  Constant6/1 -> Data Type Conversion6/1
  Constant5/1 -> Data Type Conversion5/1
  Constant4/1 -> Data Type Conversion4/1
  Constant3/1 -> Data Type Conversion3/1
  Constant2/1 -> Data Type Conversion2/1
  Constant1/1 -> Data Type Conversion1/1
  Constant12/1 -> Data Type Conversion/1
  Data Type Conversion/1 -> statusword/1
  Data Type Conversion10/1 -> "[fromSomanetToCelsius]"/1
  Data Type Conversion9/1 -> opMode/1
  Data Type Conversion8/1 -> "[fromADCtoAmp]1"/1
  Data Type Conversion7/1 -> "[fromADCtoAmp]"/1
  Data Type Conversion6/1 -> error/1
  Data Type Conversion5/1 -> tuningStatus/1
  Data Type Conversion4/1 -> userMISO/1
  Data Type Conversion3/1 -> "[frommNmToNm]"/1
  Data Type Conversion2/1 -> "[fromRPMToRad/s]"/1
  Data Type Conversion11/1 -> timestamp/1
  "[fromSomanetToCelsius]"/1 -> statusTemperature/1
  "[fromADCtoAmp]1"/1 -> statusPhaseCurrentC/1
  "[fromADCtoAmp]"/1 -> statusPhaseCurrentB/1
  "[frommNmToNm]"/1 -> actualTorque/1
  "[fromRPMToRad/s]"/1 -> actualVelocity/1
  Constant16/1 -> "[fromTicksToRad]1"/2
  "[fromTicksToRad]1"/1 -> actualMotorAngle/1
  Data Type Conversion12/1 -> "[fromTicksToRad]1"/1
  "[fromRPMToRad/s]1"/1 -> actualMotorVelocity/1
  Constant17/1 -> Degrees to Radians/1
  FromTicksToJointRad/1 -> actualAngle/1
  Data Type Conversion1/1 -> FromTicksToJointRad/1
  Constant/1 -> FromTicksToJointRad/2

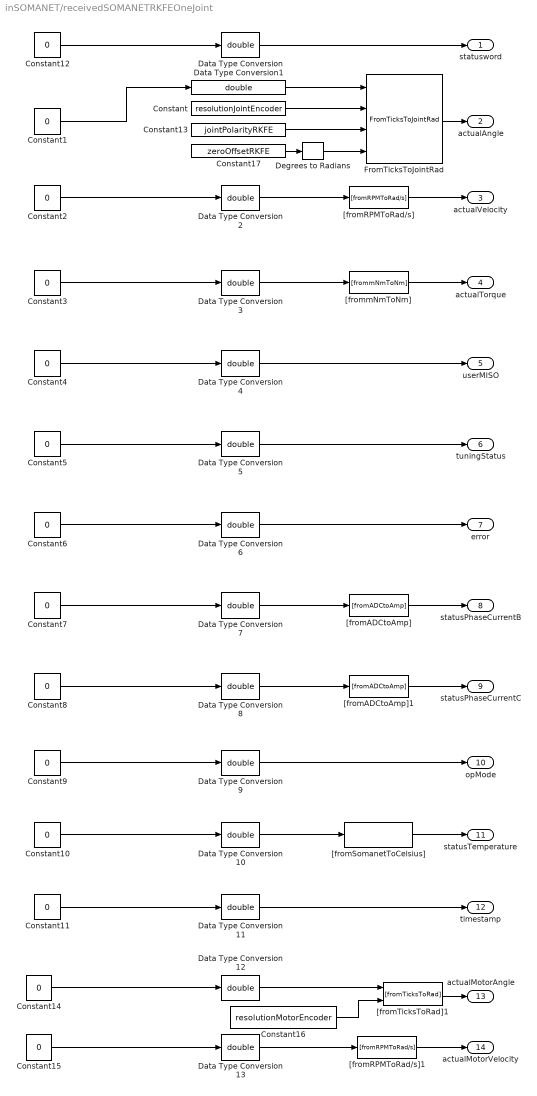
== system inSOMANET/receivedSOMANETRKFEOneJoint ==
  Constant : Constant  Value=resolutionJointEncoder
  Constant{1..12,14..15} (14 alike) : Constant  Value=0
  Constant13 : Constant  Value=jointPolarityRKFE
  Constant16 : Constant  Value=resolutionMotorEncoder
  Constant17 : Constant  Value=zeroOffsetRKFE  SampleTime=-1
  Data Type Conversion{,1..13} (14 alike) : DataTypeConversion  OutDataTypeStr=double
  Degrees to Radians : simulink_extras/Transformations/Degrees to Radians
  FromTicksToJointRad : ConversionsLibrary/FromTicksToJointRad
  "[fromADCtoAmp]" : ConversionsLibrary/[fromADCtoAmp]
  "[fromADCtoAmp]1" : ConversionsLibrary/[fromADCtoAmp]
  "[fromRPMToRad/s]" : ConversionsLibrary/[fromRPMToRad//s]
  "[fromRPMToRad/s]1" : ConversionsLibrary/[fromRPMToRad//s]
  "[fromSomanetToCelsius]" : ConversionsLibrary/[fromSomanetToCelsius]
  "[fromTicksToRad]1" : ConversionsLibrary/[fromTicksToRad]
  "[frommNmToNm]" : ConversionsLibrary/[frommNmToNm]
  statusword : Outport
  actualAngle : Outport  Port=2
  actualVelocity : Outport  Port=3
  actualTorque : Outport  Port=4
  userMISO : Outport  Port=5
  tuningStatus : Outport  Port=6
  error : Outport  Port=7
  statusPhaseCurrentB : Outport  Port=8
  statusPhaseCurrentC : Outport  Port=9
  opMode : Outport  Port=10
  statusTemperature : Outport  Port=11
  timestamp : Outport  Port=12
  actualMotorAngle : Outport  Port=13
  actualMotorVelocity : Outport  Port=14
  wires:
  Constant15/1 -> Data Type Conversion13/1
  Data Type Conversion13/1 -> "[fromRPMToRad/s]1"/1
  Constant14/1 -> Data Type Conversion12/1
  Constant11/1 -> Data Type Conversion11/1
  Constant10/1 -> Data Type Conversion10/1
  Constant9/1 -> Data Type Conversion9/1
  Constant8/1 -> Data Type Conversion8/1
  Constant7/1 -> Data Type Conversion7/1
  Constant6/1 -> Data Type Conversion6/1
  Constant5/1 -> Data Type Conversion5/1
  Constant4/1 -> Data Type Conversion4/1
  Constant3/1 -> Data Type Conversion3/1
  Constant2/1 -> Data Type Conversion2/1
  Constant12/1 -> Data Type Conversion/1
  Data Type Conversion/1 -> statusword/1
  Data Type Conversion10/1 -> "[fromSomanetToCelsius]"/1
  Data Type Conversion9/1 -> opMode/1
  Data Type Conversion8/1 -> "[fromADCtoAmp]1"/1
  Data Type Conversion7/1 -> "[fromADCtoAmp]"/1
  Data Type Conversion6/1 -> error/1
  Data Type Conversion5/1 -> tuningStatus/1
  Data Type Conversion4/1 -> userMISO/1
  Data Type Conversion3/1 -> "[frommNmToNm]"/1
  Data Type Conversion2/1 -> "[fromRPMToRad/s]"/1
  Data Type Conversion11/1 -> timestamp/1
  "[fromSomanetToCelsius]"/1 -> statusTemperature/1
  "[fromADCtoAmp]1"/1 -> statusPhaseCurrentC/1
  "[fromADCtoAmp]"/1 -> statusPhaseCurrentB/1
  "[frommNmToNm]"/1 -> actualTorque/1
  "[fromRPMToRad/s]"/1 -> actualVelocity/1
  Constant16/1 -> "[fromTicksToRad]1"/2
  "[fromTicksToRad]1"/1 -> actualMotorAngle/1
  Data Type Conversion12/1 -> "[fromTicksToRad]1"/1
  "[fromRPMToRad/s]1"/1 -> actualMotorVelocity/1
  Constant17/1 -> Degrees to Radians/1
  Degrees to Radians/1 -> FromTicksToJointRad/4
  Data Type Conversion1/1 -> FromTicksToJointRad/1
  Constant/1 -> FromTicksToJointRad/2
  Constant13/1 -> FromTicksToJointRad/3
  FromTicksToJointRad/1 -> actualAngle/1
  Constant1/1 -> Data Type Conversion1/1
